simulink model "subsystem_mask_test"  (Simulink 9.0)
settings: Solver=ode3  StartTime=0.0  StopTime=10.0  FixedStep=0.200000  RelTol=1e-3  EnableMultiTasking=on
libraries: simulink x1
settings Model: SuppressorTable=22 serialization::archive 11 0 6 0 0 0 0 0  Creator=arnaud  LastModifiedBy=hbourbou
settings DataIOCC: LimitDataPoints=on  SaveFormat=StructureWithTime  SignalLoggingSaveFormat=ModelDataLogs
settings OptimizationCC: ExpressionDepthLimit=2147483647
settings DebuggingCC: SolverPrmCheckMsg=warning  FcnCallInpInsideContextMsg=warning  StateNameClashWarn=warning
settings GRTTargetCC: GeneratePreprocessorConditionals=Disable all  CombineOutputUpdateFcns=off  GRTInterface=on
settings ConfigComp: CovSFcnEnable=off

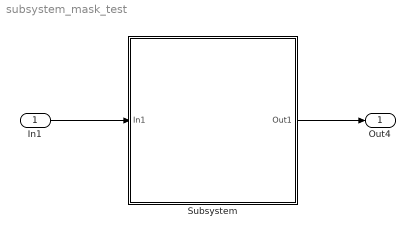
== system subsystem_mask_test ==
  In1 : Inport  PortDimensions=1
  Subsystem : Subsystem  TreatAsAtomicUnit=on
      mask Display: image('plane.jpg')
  Out4 : Outport
  wires:
  In1/1 -> Subsystem/1(In1)
  Subsystem/1(Out1) -> Out4/1

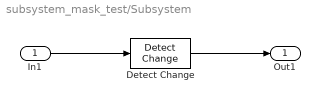
== system subsystem_mask_test/Subsystem ==
  In1 : Inport
  Detect Change : simulink/Logic and Bit Operations/Detect Change  vinit=0  InputProcessing=Inherited  OutDataTypeStr=boolean
  Out1 : Outport
  wires:
  In1/1 -> Detect Change/1
  Detect Change/1 -> Out1/1
